simulink model "nms_3Dmodel_inv_wAnkleCPG"  (R2016b)
settings: Solver=ode3  StartTime=0.0  StopTime=tend  FixedStep=ts  RelTol=1e-3  EnableMultiTasking=on
InitFcn:
  | runScripts_inv;
values from neighbouring files (symbols this model uses):
  c = 0.05    [IID_nms_MechInit.m]    (also in nms_MechInit.m)
  c_jointstop = 0.3 / (pi/180)    (= 17.1887338539)    [IID_nms_MechInit.m]    (also in nms_MechInit.m)
  CPG_On = 1    [setCPGPar.m]    (also in setCPGPar_inv.m)
  CtrlPar_FP = [alpha0 alpha_cd alpha_cv]    [setCtrlPar.m]
  CtrlPar_FP_R = [R_hipR0 R_hipR_cd R_hipR_cv]    [setCtrlPar.m]
  CtrlPar_LL = l_clr    [setCtrlPar.m]
  CtrlPar_St = [StPreStim St_M1 St_M2 St_M3 St_M4 St_M5 St_M11]    [setCtrlPar.m]
  CtrlPar_St_R = [R_StPreStim R_St_M1 R_St_M3 R_St_M4]    [setCtrlPar.m]
  CtrlPar_Sw = [SwPreStim SwPhasePari SwPhaseParii SwCtrlPar_H SwCtrlPar_A      SwCtrlPar_Ki SwCtrlPar_Kii SwCtrlPar_Kiii SwCtrlPar_StP]    [setCtrlPar.m]
  CtrlPar_Sw_R = [R_SwPreStim R_Sw_M6]    [setCtrlPar.m]
  CtrlPar_theta0 = parBlCtrl(1)      *1*pi/180    [setCtrlPar.m]
  CtrlPar_Tr = [Tr_St_sup Tr_Sw]    [setCtrlPar.m]
  CtrlPar_Tr_R = [R_Tr_St_sup R_Tr_Sw]    [setCtrlPar.m]
  eref = 0.04    [IID_nms_MechInit.m]    (also in nms_MechInit.m)
  FmaxBFSH = 350    [nms_MechInit.m]
  FmaxGAS = 1500    [IID_nms_MechInit.m]    (also in nms_MechInit.m)
  FmaxGLU = 1500    [IID_nms_MechInit.m]    (also in nms_MechInit.m)
  FmaxHAB = 3000    [nms_MechInit.m]
  FmaxHAD = 4500    [nms_MechInit.m]
  FmaxHAM = 3000    [IID_nms_MechInit.m]    (also in nms_MechInit.m)
  FmaxHFL = 2000    [IID_nms_MechInit.m]    (also in nms_MechInit.m)
  FmaxRF = 1200    [nms_MechInit.m]
  FmaxSOL = 4000    [IID_nms_MechInit.m]    (also in nms_MechInit.m)
  FmaxTA = 800    [IID_nms_MechInit.m]    (also in nms_MechInit.m)
  FmaxVAS = 6000    [IID_nms_MechInit.m]    (also in nms_MechInit.m)
  init_a_tgt = 70*pi/180    (= 1.2217304764)    [setInitPar.m]
  init_a_tgtR = 90*pi/180    (= 1.57079632679)    [setInitPar.m]
  K = 5    [IID_nms_MechInit.m]    (also in nms_MechInit.m)
  leg_l = [D12_T D12_S]    [nms_MechInit.m]
  LongDelay = 0.020    (= 0.02)    [IID_setCtrlPar.m]    (also in nms_MechInit.m = 0.01)
  LongLoopDelay = 0.030    (= 0.03)    [nms_MechInit.m]
  loptBFSH = 0.12    [nms_MechInit.m]
  loptGAS = 0.05    [IID_nms_MechInit.m]    (also in nms_MechInit.m)
  loptGLU = 0.11    [IID_nms_MechInit.m]    (also in nms_MechInit.m)
  loptHAB = 0.09    [nms_MechInit.m]
  loptHAD = 0.10    (= 0.1)    [nms_MechInit.m]
  loptHAM = 0.10    (= 0.1)    [IID_nms_MechInit.m]    (also in nms_MechInit.m)
  loptHFL = 0.11    [IID_nms_MechInit.m]    (also in nms_MechInit.m)
  loptRF = 0.08    [nms_MechInit.m]
  loptSOL = 0.04    [IID_nms_MechInit.m]    (also in nms_MechInit.m)
  loptTA = 0.06    [IID_nms_MechInit.m]    (also in nms_MechInit.m)
  loptVAS = 0.08    [IID_nms_MechInit.m]    (also in nms_MechInit.m)
  lslackBFSH = 0.10    (= 0.1)    [nms_MechInit.m]
  lslackGAS = 0.40    (= 0.4)    [IID_nms_MechInit.m]    (also in nms_MechInit.m)
  lslackGLU = 0.13    [IID_nms_MechInit.m]    (also in nms_MechInit.m)
  lslackHAB = 0.07    [nms_MechInit.m]
  lslackHAD = 0.18    [nms_MechInit.m]
  lslackHAM = 0.31    [IID_nms_MechInit.m]    (also in nms_MechInit.m)
  lslackHFL = 0.10    (= 0.1)    [IID_nms_MechInit.m]    (also in nms_MechInit.m)
  lslackRF = 0.35    [nms_MechInit.m]
  lslackSOL = 0.26    [IID_nms_MechInit.m]    (also in nms_MechInit.m)
  lslackTA = 0.24    [IID_nms_MechInit.m]    (also in nms_MechInit.m)
  lslackVAS = 0.23    [IID_nms_MechInit.m]    (also in nms_MechInit.m)
  massBFSH = 2    [nms_MechInit.m]
  massGAS = 0.45    [IID_nms_MechInit.m]    (also in nms_MechInit.m)
  massGLU = 1.4    [IID_nms_MechInit.m]    (also in nms_MechInit.m)
  massHAB = 1.145    [nms_MechInit.m]
  massHAD = 1.91    [nms_MechInit.m]
  massHAM = 1.82    [IID_nms_MechInit.m]    (also in nms_MechInit.m)
  massHFL = 1.87    [IID_nms_MechInit.m]    (also in nms_MechInit.m)
  massRF = 1    [nms_MechInit.m]
  massSOL = 1.36    [IID_nms_MechInit.m]    (also in nms_MechInit.m)
  massTA = 0.29    [IID_nms_MechInit.m]    (also in nms_MechInit.m)
  massVAS = 2.91    [IID_nms_MechInit.m]    (also in nms_MechInit.m)
  MidDelay = 0.010    (= 0.01)    [IID_setCtrlPar.m]    (also in nms_MechInit.m = 0.005)
  N = 1.5    [IID_nms_MechInit.m]    (also in cmaes_parfor.m = size(x,1); nms_MechInit.m)
  phi12_LowLimit = 70*pi/180    (= 1.2217304764)    [IID_nms_MechInit.m]    (also in nms_MechInit.m)
  phi12_UpLimit = 130*pi/180    (= 2.26892802759)    [IID_nms_MechInit.m]    (also in nms_MechInit.m)
  phi23_UpLimit = 175*pi/180    (= 3.05432619099)    [IID_nms_MechInit.m]    (also in nms_MechInit.m)
  phi34_UpLimit = 230*pi/180    (= 4.01425727959)    [IID_nms_MechInit.m]    (also in nms_MechInit.m)
  phi34R_LowLimit = -15*pi/180    (= -0.261799387799)    [nms_MechInit.m]
  phi34R_UpLimit = 50*pi/180    (= 0.872664625997)    [nms_MechInit.m]
  phimaxGASa = 110*pi/180    (= 1.91986217719)    [IID_nms_MechInit.m]    (also in nms_MechInit.m = 1.74532925199)
  phimaxGASk = 140*pi/180    (= 2.44346095279)    [IID_nms_MechInit.m]    (also in nms_MechInit.m)
  phimaxRFk = 165*pi/180    (= 2.87979326579)    [nms_MechInit.m]
  phimaxSOL = 110*pi/180    (= 1.91986217719)    [IID_nms_MechInit.m]    (also in nms_MechInit.m = 1.74532925199)
  phimaxTA = 80*pi/180    (= 1.3962634016)    [IID_nms_MechInit.m]    (also in nms_MechInit.m)
  phimaxVAS = 165*pi/180    (= 2.87979326579)    [IID_nms_MechInit.m]    (also in nms_MechInit.m)
  phirefBFSH = 160*pi/180    (= 2.79252680319)    [nms_MechInit.m]
  phirefGASa = 80*pi/180    (= 1.3962634016)    [IID_nms_MechInit.m]    (also in nms_MechInit.m)
  phirefGASk = 165*pi/180    (= 2.87979326579)    [IID_nms_MechInit.m]    (also in nms_MechInit.m)
  phirefGLU = 150*pi/180    (= 2.61799387799)    [IID_nms_MechInit.m]    (also in nms_MechInit.m = 2.09439510239)
  phirefHAB = 10*pi/180    (= 0.174532925199)    [nms_MechInit.m]
  phirefHAD = 15*pi/180    (= 0.261799387799)    [nms_MechInit.m]
  phirefHAMh = 155*pi/180    (= 2.70526034059)    [IID_nms_MechInit.m]    (also in nms_MechInit.m = 2.61799387799)
  phirefHAMk = 180*pi/180    (= 3.14159265359)    [IID_nms_MechInit.m]    (also in nms_MechInit.m)
  phirefHFL = 180*pi/180    (= 3.14159265359)    [IID_nms_MechInit.m]    (also in nms_MechInit.m = 2.79252680319)
  phirefRFh = 170*pi/180    (= 2.96705972839)    [nms_MechInit.m]
  phirefRFk = 125*pi/180    (= 2.18166156499)    [nms_MechInit.m]
  phirefSOL = 80*pi/180    (= 1.3962634016)    [IID_nms_MechInit.m]    (also in nms_MechInit.m = 1.57079632679)
  phirefTA = 110*pi/180    (= 1.91986217719)    [IID_nms_MechInit.m]    (also in nms_MechInit.m)
  phirefVAS = 125*pi/180    (= 2.18166156499)    [IID_nms_MechInit.m]    (also in nms_MechInit.m = 2.09439510239)
  phiScaleGASa = acos(rGASamin/rGASamax)/(phiminGASa-phimaxGASa)    [nms_MechInit.m]
  phiScaleGASk = acos(rGASkmin/rGASkmax)/(phiminGASk-phimaxGASk)    [nms_MechInit.m]
  phiScaleRFk = acos(rRFkmin/rRFkmax)/(phiminRFk-phimaxRFk)    [nms_MechInit.m]
  phiScaleSOL = acos(rSOLmin/rSOLmax)/(phiminSOL-phimaxSOL)    [nms_MechInit.m]
  phiScaleTA = acos(rTAmin/rTAmax)/(phiminTA-phimaxTA)    [nms_MechInit.m]
  phiScaleVAS = acos(rVASmin/rVASmax)/(phiminVAS-phimaxVAS)    [nms_MechInit.m]
  rBFSH = 0.04    [nms_MechInit.m]
  rGASamax = 0.06    [nms_MechInit.m]
  rGASkmax = 0.05    [nms_MechInit.m]
  rGLU = 0.10    (= 0.1)    [IID_nms_MechInit.m]    (also in nms_MechInit.m = 0.08)
  rHAB = 0.06    [nms_MechInit.m]
  rHAD = 0.03    [nms_MechInit.m]
  rHAMh = 0.08    [IID_nms_MechInit.m]    (also in nms_MechInit.m)
  rHAMk = 0.05    [IID_nms_MechInit.m]    (also in nms_MechInit.m)
  rHFL = 0.10    (= 0.1)    [IID_nms_MechInit.m]    (also in nms_MechInit.m = 0.08)
  rhoBFSH = 0.7    [nms_MechInit.m]
  rhoGASa = 0.7    [IID_nms_MechInit.m]    (also in nms_MechInit.m)
  rhoGASk = 0.7    [IID_nms_MechInit.m]    (also in nms_MechInit.m)
  rhoGLU = 0.5    [IID_nms_MechInit.m]    (also in nms_MechInit.m)
  rhoHAB = 0.7    [nms_MechInit.m]
  rhoHAD = 1    [nms_MechInit.m]
  rhoHAMh = 0.7    [IID_nms_MechInit.m]    (also in nms_MechInit.m = 0.5)
  rhoHAMk = 0.7    [IID_nms_MechInit.m]    (also in nms_MechInit.m = 0.5)
  rhoHFL = 0.5    [IID_nms_MechInit.m]    (also in nms_MechInit.m)
  rhoRFh = 0.3    [nms_MechInit.m]
  rhoRFk = 0.5    [nms_MechInit.m]
  rhoSOL = 0.5    [IID_nms_MechInit.m]    (also in nms_MechInit.m)
  rhoTA = 0.7    [IID_nms_MechInit.m]    (also in nms_MechInit.m)
  ... (+55 more)
libraries: simulink_extras x30, nmc x30, simulink x22, NMCCPG_Library x13, powerlib_meascontrol x5
(part 1 of 12)
settings Model: SimulationMode=accelerator  Creator=Tycho  LastModifiedBy=brugtjh
settings DataIOCC: SignalLogging=off  SignalLoggingName=logout
settings OptimizationCC: LifeSpan=inf
settings DebuggingCC: AllowSymbolicDim=off  SFUnexpectedBacktrackingDiag=warning  SFNoUnconditionalDefaultTransitionDiag=warning  SFExecutionAtInitializationDiag=none
settings ModelReferenceCC: PropagateSignalLabelsOutOfModel=off
settings GRTTargetCC: TargetLangStandard=C89/C90 (ANSI)
settings ConfigComp: CovMetricSettings=dw  CovHtmlReporting=on  CovSaveCumulativeToWorkspaceVar=on  CovSaveSingleToWorkspaceVar=on  CovExternalEMLEnable=off

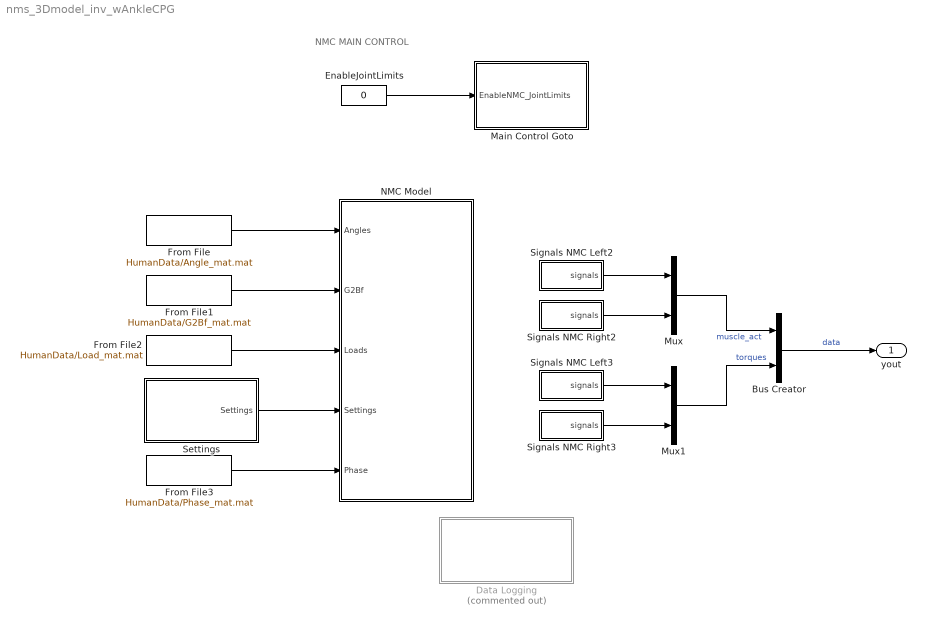
== system nms_3Dmodel_inv_wAnkleCPG ==
  note: NMC MAIN CONTROL
  Bus Creator : BusCreator  Inputs=2
  Data Logging : Subsystem  Commented=on
  EnableJointLimits : Constant  Value=0  OutDataTypeStr=double
      settings: OpenFcn=|
      | b = get_param(gcb,'value');
      | if (strcmp(b,'1')),
      |   set_param (gcb,'value','0');
      | else
      |   set_param(gcb,'value','1');
      | end;
  From File : FromFile  FileName=HumanData/Angle_mat.mat  SampleTime=0
  From File1 : FromFile  FileName=HumanData/G2Bf_mat.mat  SampleTime=0
  From File2 : FromFile  FileName=HumanData/Load_mat.mat  SampleTime=0
  From File3 : FromFile  FileName=HumanData/Phase_mat.mat  SampleTime=0
  Main Control Goto : Subsystem
  Mux : Mux  Inputs=2
  Mux1 : Mux  Inputs=2
  NMC Model : Subsystem
  Settings : Subsystem
  Signals NMC Left2 : Subsystem
  Signals NMC Left3 : Subsystem
  Signals NMC Right2 : Subsystem
  Signals NMC Right3 : Subsystem
  yout : Outport
  wires:
  Settings/1(Settings) -> NMC Model/4(Settings)
  EnableJointLimits/1 -> Main Control Goto/1(EnableNMC_JointLimits)
  From File/1 -> NMC Model/1(Angles)
  From File1/1 -> NMC Model/2(G2Bf)
  From File2/1 -> NMC Model/3(Loads)
  From File3/1 -> NMC Model/5(Phase)
  Signals NMC Right2/1(signals) -> Mux/2
  Signals NMC Left2/1(signals) -> Mux/1
  Signals NMC Left3/1(signals) -> Mux1/1
  Signals NMC Right3/1(signals) -> Mux1/2
  Mux/1 -> Bus Creator/1  "muscle_act"
  Mux1/1 -> Bus Creator/2  "torques"
  Bus Creator/1 -> yout/1  "data"

== system nms_3Dmodel_inv_wAnkleCPG/Data Logging ==
  note: Sensors
  note: Stance Info
  note: Muscle Activation
  note: Joint Torques
  note: Body Info
  note: Joint Torques (Passive)
  note: Muscle Power
  note: Angle of Attack
  Angles1 : Subsystem
  BodyInfo1 : Subsystem
  Joint Torques1 : Subsystem
  Joint TorquesPassive1 : Subsystem
  Joint TorquesTotal1 : Subsystem
  Loads1 : Subsystem
  M1 : Subsystem
  Muscle Activation2 : Subsystem
  Muscle Power1 : Subsystem
  Mux : Mux  Inputs=2
  Mux3 : Mux  Inputs=8
  Positions1 : Subsystem
  Selector2 : Selector  InputPortWidth=2  IndexOptions=Index vector (dialog)  Indices=[2]  OutputSizes=1
  Selector3 : Selector  InputPortWidth=2  IndexOptions=Index vector (dialog)  Indices=[2]  OutputSizes=1
  Sensors : Subsystem
  Signals NMC Left10 : Subsystem
  Signals NMC Left11 : Subsystem
  Signals NMC Left13 : Subsystem
  Signals NMC Left14 : Subsystem
  Signals NMC Left3 : Subsystem
  Signals NMC Left9 : Subsystem
  Signals NMC Right4 : Subsystem
  Signals NMC Right5 : Subsystem
  Signals NMC Right6 : Subsystem
  SignalsFromNMC_L1 : Subsystem  mask{LorR='L', Add=''}
      mask prompts: LorR "Right or Left"; Add "Addition"
      mask init:
      | blk = gcb;
      | set_param([gcb '/From'],'GotoTag',[LorR,'FmGLU',Add]);
      | set_param([gcb '/From1'],'GotoTag',[LorR,'FmHAM',Add]);
      | set_param([gcb '/From2'],'GotoTag',[LorR,'FmVAS',Add]);
      | set_param([gcb '/From3'],'GotoTag',[LorR,'LceBFSH',Add]);
      | set_param([gcb '/From4'],'GotoTag',[LorR,'FmGAS',Add]);
      | 
      | set_param([gcb '/From5'],'GotoTag',[LorR,'FmSOL',Add]);
      | set_param([gcb '/From6'],'GotoTag',[LorR,'LceTA',Add]);
      | set_param([gcb '/From7'],'GotoTag',[LorR,'LceRF',Add]);
      | set_param([gcb '/From8'],'GotoTag',[LorR,'VceRF',Add]);
      | set_param([gcb '/From9'],'GotoTag',[LorR,'LceHAM',Add]);
      | 
      | set_param([gcb '/From10'],'GotoTag',[LorR,'VceHAM',Add]);
      | set_param([gcb '/From11'],'GotoTag',[LorR,'VceVAS',Add]);
      | set_param([gcb '/From12'],'GotoTag',[LorR,'VceBFSH',Add]);
      | set_param([gcb '/From13'],'GotoTag',[LorR,'LceHFL',Add]);
      | set_param([gcb '/From14'],'GotoTag',[LorR,'LceGLU',Add]);
      | 
      | set_param([gcb '/From15'],'GotoTag',[LorR,'LceVAS',Add]);
      | set_param([gcb '/From16'],'GotoTag',[LorR,'FmHAB',Add]);
      | set_param([gcb '/From17'],'GotoTag',[LorR,'LceHAD',Add]);
      | set_param([gcb '/From18'],'GotoTag',[LorR,'LceHAB',Add]);
  SignalsFromNMC_L2 : Subsystem  mask{LorR='R', Add=''}
      mask prompts: LorR "Right or Left"; Add "Addition"
      mask init: same as nms_3Dmodel_inv_wAnkleCPG/Data Logging/SignalsFromNMC_L1
  StanceInfo1 : Subsystem
  Subsystem : Subsystem
  wires:
  SignalsFromNMC_L1/1(SigOut) -> Sensors/1(LC)
  SignalsFromNMC_L2/1(SigOut) -> Sensors/2(RC)
  Signals NMC Right5/1(signals) -> Muscle Activation2/2(R_MA)
  Signals NMC Left9/1(signals) -> Muscle Activation2/1(L_MA)
  Signals NMC Left10/1(signals) -> Joint TorquesTotal1/1(LTor)
  Signals NMC Right6/1(signals) -> Joint TorquesTotal1/2(RTor)
  Angles1/1(Angles) -> BodyInfo1/1(Angles)
  Positions1/1(Positions) -> BodyInfo1/2(Postitions)
  [LStance] -> StanceInfo1/1(LStance)
  [RStance] -> StanceInfo1/2(RStance)
  Loads1/1(Loads) -> BodyInfo1/3(Loads)
  [rotTrunk] -> Mux/1
  [theta] -> Mux/2
  Signals NMC Left11/1(signals) -> Joint TorquesPassive1/1(LTor)
  Signals NMC Right4/1(signals) -> Joint TorquesPassive1/2(RTor)
  Selector2/1 -> Mux3/1
  [front_dv_L] -> Selector2/1
  [L_M_TOT] -> Mux3/5
  [R_M_TOT] -> Mux3/6
  [L_M11_TOT] -> Mux3/3
  [R_M11_TOT] -> Mux3/4
  [front_dv_R] -> Selector3/1
  Selector3/1 -> Mux3/2
  Signals NMC Left13/1(signals) -> Muscle Power1/2(R_MA)
  Signals NMC Left14/1(signals) -> Muscle Power1/1(L_MA)
  Mux3/1 -> M1/1(M11)
  Mux/1 -> Subsystem/1(RotTrunk)
  [M11_Control] -> Mux3/8
  Signals NMC Left3/1(Target) -> Joint Torques1/1(Target)
  [front_v_est] -> Mux3/7

== system nms_3Dmodel_inv_wAnkleCPG/Main Control Goto ==
  EnableNMC_JointLimits : Inport
  tag scope: DisableNMC_JointLimitsIn=global
  wires:
  EnableNMC_JointLimits/1 -> [DisableNMC_JointLimitsIn]

== system nms_3Dmodel_inv_wAnkleCPG/NMC Model ==
  note: Data Distribution
  note: NMS model based on:
      | The nms_3Dmodel is a neuromechanical model of 3D human locomotion.
      | The details of the model are explained in:
      | S Song and H Geyer. "A neural circuitry that emphasizes spinal feedback
      | generates diverse behaviours of human locomotion." The Journal of physiology (2015).
      |
      | Muscle Actuation Layer:
      | The joints are actuated by 11 Hill-type muscles per leg.
      |
      | Neural Control Layer:
      | The muscles are controlled by local reflexes.
      |
      | Higher Control Layer:
      | The reflex pathways are modulated by the higher layer control.
  note: Neuromuscular Locomotion Model for Lopes
  note: DataStore for CPG
  Angles : Inport
  G2Bf : Inport  Port=2
  Loads : Inport  Port=3
  Settings : Inport  Port=4
  Phase : Inport  Port=5
  CPG : Subsystem
  Demux : Demux  Outputs=8
  Demux1 : Demux
  Demux2 : Demux  Outputs=2
  Demux4 : Demux
  Higher Control Layer (Supra Spinal Control) : Subsystem
  Muscle Actuation Layer : Subsystem
  Neural Control Layer (Spinal Cord Control) : Subsystem
  Rounding Function : Rounding  Operator=round
  Selector : Selector  InputPortWidth=12  IndexOptions=Index vector (dialog)  Indices=[1:4]  OutputSizes=1
  Selector1 : Selector  InputPortWidth=12  IndexOptions=Index vector (dialog)  Indices=[5:12]  OutputSizes=1
  data_l_st_freq : DataStoreMemory  DataStoreName=Freq_Ph1  ReadBeforeWriteMsg=warning  WriteAfterWriteMsg=warning  WriteAfterReadMsg=warning  InitialValue=FreqPL_Ph1  VectorParams1D=off  ShowAdditionalParam=off
  data_l_st_freq1 : DataStoreMemory  DataStoreName=Freq_Ph3  ReadBeforeWriteMsg=warning  WriteAfterWriteMsg=warning  WriteAfterReadMsg=warning  InitialValue=FreqPL_Ph3  VectorParams1D=off  ShowAdditionalParam=off
  data_l_st_shape : DataStoreMemory  DataStoreName=Shape_Ph1  ReadBeforeWriteMsg=warning  WriteAfterWriteMsg=warning  WriteAfterReadMsg=warning  InitialValue=ShapePL_Ph1  VectorParams1D=off  ShowAdditionalParam=off
  data_l_st_shape1 : DataStoreMemory  DataStoreName=Shape_Ph3  ReadBeforeWriteMsg=warning  WriteAfterWriteMsg=warning  WriteAfterReadMsg=warning  InitialValue=ShapePL_Ph3  VectorParams1D=off  ShowAdditionalParam=off
  data_l_sw_freq : DataStoreMemory  DataStoreName=Freq_Ph2  ReadBeforeWriteMsg=warning  WriteAfterWriteMsg=warning  WriteAfterReadMsg=warning  InitialValue=FreqPL_Ph2  VectorParams1D=off  ShowAdditionalParam=off
  data_l_sw_freq1 : DataStoreMemory  DataStoreName=Freq_Ph4  ReadBeforeWriteMsg=warning  WriteAfterWriteMsg=warning  WriteAfterReadMsg=warning  InitialValue=FreqPL_Ph4  VectorParams1D=off  ShowAdditionalParam=off
  data_l_sw_shape : DataStoreMemory  DataStoreName=Shape_Ph2  ReadBeforeWriteMsg=warning  WriteAfterWriteMsg=warning  WriteAfterReadMsg=warning  InitialValue=ShapePL_Ph2  VectorParams1D=off  ShowAdditionalParam=off
  data_l_sw_shape1 : DataStoreMemory  DataStoreName=Shape_Ph4  ReadBeforeWriteMsg=warning  WriteAfterWriteMsg=warning  WriteAfterReadMsg=warning  InitialValue=ShapePL_Ph4  VectorParams1D=off  ShowAdditionalParam=off
  etc : Subsystem
  tag scope: DisableNMC_JointLimits=global, LLLoad=global, Lphi12dphi12=global, Lphi23dphi23=global, Lphi34dphi34=global, Lphi34dphi34R=global, RLLoad=global, Rphi12dphi12=global, Rphi23dphi23=global, Rphi34dphi34=global, Rphi34dphi34R=global, dtheta=global, dthetaR=global, front_dv_L=global, front_dv_R=global, phase=global, side_dv_L=global, side_dv_R=global, theta=global, thetaR=global
  wires:
  Settings/1 -> [DisableNMC_JointLimits]
  Phase/1 -> Rounding Function/1
  Demux2/2 -> [RLLoad]
  Demux2/1 -> [LLLoad]
  Loads/1 -> Demux2/1
  G2Bf/1 -> Selector1/1, Selector/1
  Demux/4 -> [Lphi12dphi12]
  Demux/3 -> [Lphi23dphi23]
  Demux/2 -> [Lphi34dphi34R]
  Demux/8 -> [Rphi12dphi12]
  Demux/7 -> [Rphi23dphi23]
  Demux/6 -> [Rphi34dphi34R]
  Demux/5 -> [Rphi34dphi34]
  Demux/1 -> [Lphi34dphi34]
  Angles/1 -> Demux/1
  Demux4/1 -> [front_dv_L]
  Demux4/2 -> [front_dv_R]
  Demux4/3 -> [side_dv_L]
  Demux4/4 -> [side_dv_R]
  Demux1/4 -> [dthetaR]
  Demux1/3 -> [thetaR]
  Demux1/2 -> [dtheta]
  Demux1/1 -> [theta]
  Selector/1 -> Demux1/1
  Selector1/1 -> Demux4/1
  Rounding Function/1 -> [phase]

== system nms_3Dmodel_inv_wAnkleCPG/Settings ==
  Settings : Outport
  wires:
  [DisableNMC_JointLimitsIn] -> Settings/1

== system nms_3Dmodel_inv_wAnkleCPG/Signals NMC Left2 ==
  Mux : Mux  Inputs=11
  signals : Outport
  wires:
  Mux/1 -> signals/1
  [LStimHFL] -> Mux/1
  [LStimGLU] -> Mux/9
  [LStimVAS] -> Mux/3
  [LStimBFSH] -> Mux/7
  [LStimHAD] -> Mux/11
  [LStimSOL] -> Mux/5
  [LStimHAB] -> Mux/10
  [LStimHAM] -> Mux/8
  [LStimGAS] -> Mux/6
  [LStimTA] -> Mux/4
  [LStimRF] -> Mux/2

== system nms_3Dmodel_inv_wAnkleCPG/Signals NMC Left3 ==
  Mux : Mux
  signals : Outport
  wires:
  Mux/1 -> signals/1
  [LM34] -> Mux/1
  [LM23] -> Mux/3
  [LM12] -> Mux/4
  [LM34R] -> Mux/2

== system nms_3Dmodel_inv_wAnkleCPG/Signals NMC Right2 ==
  Mux : Mux  Inputs=11
  signals : Outport
  wires:
  [RStimRF] -> Mux/2
  [RStimTA] -> Mux/4
  [RStimGAS] -> Mux/6
  [RStimHAM] -> Mux/8
  [RStimHAB] -> Mux/10
  [RStimSOL] -> Mux/5
  [RStimHAD] -> Mux/11
  [RStimBFSH] -> Mux/7
  [RStimVAS] -> Mux/3
  [RStimGLU] -> Mux/9
  [RStimHFL] -> Mux/1
  Mux/1 -> signals/1

== system nms_3Dmodel_inv_wAnkleCPG/Signals NMC Right3 ==
  Mux : Mux
  signals : Outport
  wires:
  Mux/1 -> signals/1
  [RM34] -> Mux/1
  [RM23] -> Mux/3
  [RM12] -> Mux/4
  [RM34R] -> Mux/2

== system nms_3Dmodel_inv_wAnkleCPG/Data Logging/Angles1 ==
  Mux : Mux  Inputs=8
  Angles : Outport
  wires:
  [Rphi12dphi12] -> Mux/8
  [Lphi34dphi34] -> Mux/1
  [Rphi23dphi23] -> Mux/7
  [Lphi23dphi23] -> Mux/3
  [Rphi34dphi34R] -> Mux/6
  [Lphi34dphi34R] -> Mux/2
  [Lphi12dphi12] -> Mux/4
  [Rphi34dphi34] -> Mux/5
  Mux/1 -> Angles/1

== system nms_3Dmodel_inv_wAnkleCPG/Data Logging/BodyInfo1 ==
  Angles : Inport
  Postitions : Inport  Port=2
  Loads : Inport  Port=3
  Mux1 : Mux  Inputs=3
  To File8 : ToFile  Filename=Records/BodyInfo
  wires:
  Loads/1 -> Mux1/3
  Postitions/1 -> Mux1/2
  Mux1/1 -> To File8/1
  Angles/1 -> Mux1/1

== system nms_3Dmodel_inv_wAnkleCPG/Data Logging/Joint Torques1 ==
  Target : Inport
  To File12 : ToFile  Filename=Records/TargetAngle
  wires:
  Target/1 -> To File12/1

== system nms_3Dmodel_inv_wAnkleCPG/Data Logging/Joint TorquesPassive1 ==
  LTor : Inport
  RTor : Inport  Port=2
  To File12 : ToFile  Filename=Records/L_Tor_Passive
  To File9 : ToFile  Filename=Records/R_Tor_Passvie
  wires:
  RTor/1 -> To File9/1
  LTor/1 -> To File12/1

== system nms_3Dmodel_inv_wAnkleCPG/Data Logging/Joint TorquesTotal1 ==
  LTor : Inport
  RTor : Inport  Port=2
  To File12 : ToFile  Filename=Records/L_Tor
  To File9 : ToFile  Filename=Records/R_Tor
  wires:
  LTor/1 -> To File12/1
  RTor/1 -> To File9/1

== system nms_3Dmodel_inv_wAnkleCPG/Data Logging/Loads1 ==
  Mux : Mux  Inputs=2
  Loads : Outport
  wires:
  [LLLoad] -> Mux/2
  [RLLoad] -> Mux/1
  Mux/1 -> Loads/1

== system nms_3Dmodel_inv_wAnkleCPG/Data Logging/M1 ==
  M11 : Inport
  To File2 : ToFile  Filename=Records/M11
  wires:
  M11/1 -> To File2/1

== system nms_3Dmodel_inv_wAnkleCPG/Data Logging/Muscle Activation2 ==
  L_MA : Inport
  R_MA : Inport  Port=2
  To File1 : ToFile  Filename=Records/R_MA
  To File5 : ToFile  Filename=Records/L_MA
  wires:
  L_MA/1 -> To File5/1
  R_MA/1 -> To File1/1

== system nms_3Dmodel_inv_wAnkleCPG/Data Logging/Muscle Power1 ==
  L_MA : Inport
  R_MA : Inport  Port=2
  To File1 : ToFile  Filename=Records/R_Power
  To File5 : ToFile  Filename=Records/L_Power
  wires:
  L_MA/1 -> To File5/1
  R_MA/1 -> To File1/1

== system nms_3Dmodel_inv_wAnkleCPG/Data Logging/Positions1 ==
  Mux : Mux  Inputs=19
  Positions : Outport
  wires:
  [xyzRMBall] -> Mux/19
  [xyzRLBall] -> Mux/18
  [xyzRMHeel] -> Mux/17
  [xyzRLHeel] -> Mux/16
  [xyzLMBall] -> Mux/15
  [xyzLLBall] -> Mux/14
  [xyzLMHeel] -> Mux/13
  [xyzLLHeel] -> Mux/12
  [xyzTrunk] -> Mux/11
  [dxyzHAT] -> Mux/2
  [xyzHAT] -> Mux/1
  [dxyzRHip] -> Mux/10
  [xyzRHip] -> Mux/9
  [xyzLAnkle] -> Mux/3
  [xyzRKnee] -> Mux/8
  [dxyzLHip] -> Mux/6
  [xyzLHip] -> Mux/5
  [xyzLKnee] -> Mux/4
  [xyzRAnkle] -> Mux/7
  Mux/1 -> Positions/1

== system nms_3Dmodel_inv_wAnkleCPG/Data Logging/Sensors ==
  LC : Inport
  RC : Inport  Port=2
  To File19 : ToFile  Filename=Records/L_Clean
  To File20 : ToFile  Filename=Records/R_Clean
  wires:
  RC/1 -> To File20/1
  LC/1 -> To File19/1

== system nms_3Dmodel_inv_wAnkleCPG/Data Logging/Signals NMC Left10 ==
  Mux : Mux
  signals : Outport
  wires:
  [LM34R] -> Mux/2
  [LM12] -> Mux/4
  [LM23] -> Mux/3
  [LM34] -> Mux/1
  Mux/1 -> signals/1

== system nms_3Dmodel_inv_wAnkleCPG/Data Logging/Signals NMC Left11 ==
  Mux : Mux
  signals : Outport
  wires:
  Mux/1 -> signals/1
  [LHipStop] -> Mux/1
  [LKneeStop] -> Mux/3
  [LAnkleStop] -> Mux/4
  [LHipRStop] -> Mux/2

== system nms_3Dmodel_inv_wAnkleCPG/Data Logging/Signals NMC Left13 ==
  Mux : Mux  Inputs=11
  signals : Outport
  wires:
  Mux/1 -> signals/1
  [REnergyHFL] -> Mux/1
  [REnergyGLU] -> Mux/9
  [REnergyVAS] -> Mux/3
  [REnergyBFSH] -> Mux/7
  [REnergyHAD] -> Mux/11
  [REnergySOL] -> Mux/5
  [REnergyHAB] -> Mux/10
  [REnergyHAM] -> Mux/8
  [REnergyGAS] -> Mux/6
  [REnergyTA] -> Mux/4
  [REnergyRF] -> Mux/2

== system nms_3Dmodel_inv_wAnkleCPG/Data Logging/Signals NMC Left14 ==
  Mux : Mux  Inputs=11
  signals : Outport
  wires:
  [LEnergyRF] -> Mux/2
  [LEnergyTA] -> Mux/4
  [LEnergyGAS] -> Mux/6
  [LEnergyHAM] -> Mux/8
  [LEnergyHAB] -> Mux/10
  [LEnergySOL] -> Mux/5
  [LEnergyHAD] -> Mux/11
  [LEnergyBFSH] -> Mux/7
  [LEnergyVAS] -> Mux/3
  [LEnergyGLU] -> Mux/9
  [LEnergyHFL] -> Mux/1
  Mux/1 -> signals/1

== system nms_3Dmodel_inv_wAnkleCPG/Data Logging/Signals NMC Left3 ==
  Mux : Mux
  Target : Outport
  wires:
  Mux/1 -> Target/1
  [Lalpha_tgt] -> Mux/1
  [LhipR_tgt] -> Mux/3
  [RhipR_tgt] -> Mux/4
  [Ralpha_tgt] -> Mux/2

== system nms_3Dmodel_inv_wAnkleCPG/Data Logging/Signals NMC Left9 ==
  Mux : Mux  Inputs=11
  signals : Outport
  wires:
  [LStimRF] -> Mux/2
  [LStimTA] -> Mux/4
  [LStimGAS] -> Mux/6
  [LStimHAM] -> Mux/8
  [LStimHAB] -> Mux/10
  [LStimSOL] -> Mux/5
  [LStimHAD] -> Mux/11
  [LStimBFSH] -> Mux/7
  [LStimVAS] -> Mux/3
  [LStimGLU] -> Mux/9
  [LStimHFL] -> Mux/1
  Mux/1 -> signals/1

== system nms_3Dmodel_inv_wAnkleCPG/Data Logging/Signals NMC Right4 ==
  Mux : Mux
  signals : Outport
  wires:
  Mux/1 -> signals/1
  [RHipStop] -> Mux/1
  [RKneeStop] -> Mux/3
  [RAnkleStop] -> Mux/4
  [RHipStopR] -> Mux/2

== system nms_3Dmodel_inv_wAnkleCPG/Data Logging/Signals NMC Right5 ==
  Mux : Mux  Inputs=11
  signals : Outport
  wires:
  Mux/1 -> signals/1
  [RStimHFL] -> Mux/1
  [RStimGLU] -> Mux/9
  [RStimVAS] -> Mux/3
  [RStimBFSH] -> Mux/7
  [RStimHAD] -> Mux/11
  [RStimSOL] -> Mux/5
  [RStimHAB] -> Mux/10
  [RStimHAM] -> Mux/8
  [RStimGAS] -> Mux/6
  [RStimTA] -> Mux/4
  [RStimRF] -> Mux/2

== system nms_3Dmodel_inv_wAnkleCPG/Data Logging/Signals NMC Right6 ==
  Mux : Mux
  signals : Outport
  wires:
  [RM34R] -> Mux/2
  [RM12] -> Mux/4
  [RM23] -> Mux/3
  [RM34] -> Mux/1
  Mux/1 -> signals/1

== system nms_3Dmodel_inv_wAnkleCPG/Data Logging/SignalsFromNMC_L1 ==
  Mux1 : Mux  Inputs=19
  SigOut : Outport
  wires:
  [LLceVAS] -> Mux1/16
  [LVceHAM] -> Mux1/11
  Mux1/1 -> SigOut/1
  [LVceVAS] -> Mux1/12
  [LLceRF] -> Mux1/8
  [LLceGLU] -> Mux1/15
  [LFmGAS] -> Mux1/5
  [LVceBFSH] -> Mux1/13
  [LLceHAD] -> Mux1/18
  [LVceRF] -> Mux1/9
  [LLceBFSH] -> Mux1/4
  [LFmGLU] -> Mux1/1
  [LFmSOL] -> Mux1/6
  [LLceHFL] -> Mux1/14
  [LFmVAS] -> Mux1/3
  [LLceTA] -> Mux1/7
  [LFmHAM] -> Mux1/2
  [LLceHAM] -> Mux1/10
  [LFmHAB] -> Mux1/17
  [LLceHAB] -> Mux1/19

== system nms_3Dmodel_inv_wAnkleCPG/Data Logging/SignalsFromNMC_L2 ==
  Mux1 : Mux  Inputs=19
  SigOut : Outport
  wires:
  [RLceHAB] -> Mux1/19
  [RFmHAB] -> Mux1/17
  [RLceHAM] -> Mux1/10
  [RFmHAM] -> Mux1/2
  [RLceTA] -> Mux1/7
  [RFmVAS] -> Mux1/3
  [RLceHFL] -> Mux1/14
  [RFmSOL] -> Mux1/6
  [RFmGLU] -> Mux1/1
  [RLceBFSH] -> Mux1/4
  [RVceRF] -> Mux1/9
  [RLceHAD] -> Mux1/18
  [RVceBFSH] -> Mux1/13
  [RFmGAS] -> Mux1/5
  [RLceGLU] -> Mux1/15
  [RLceRF] -> Mux1/8
  [RVceVAS] -> Mux1/12
  Mux1/1 -> SigOut/1
  [RVceHAM] -> Mux1/11
  [RLceVAS] -> Mux1/16

== system nms_3Dmodel_inv_wAnkleCPG/Data Logging/StanceInfo1 ==
  LStance : Inport
  RStance : Inport  Port=2
  Mux4 : Mux  Inputs=2
  To File4 : ToFile  Filename=Records/StanceSig
  wires:
  LStance/1 -> Mux4/1
  RStance/1 -> Mux4/2
  Mux4/1 -> To File4/1

== system nms_3Dmodel_inv_wAnkleCPG/Data Logging/Subsystem ==
  RotTrunk : Inport
  To File8 : ToFile  Filename=Records/rotTrunk
  wires:
  RotTrunk/1 -> To File8/1

== system nms_3Dmodel_inv_wAnkleCPG/NMC Model/CPG ==
  note: CPG State Observer
      | Learning Center
      | Learns the signals of all sensors
      | If signals are prelearned, only loads the signals
      |
      | CPG Output
      | Estimates rate of change (roc at all instances of various time model
      | Becomes active after signals are saved or loaded
      |
      | Saver
      | Saves signals to workspace after learning is done
      |
      | Etc
      | Creates signals necessary in CPG model
  CPG Output : Subsystem
  Etc : Subsystem
  Learning center : Subsystem

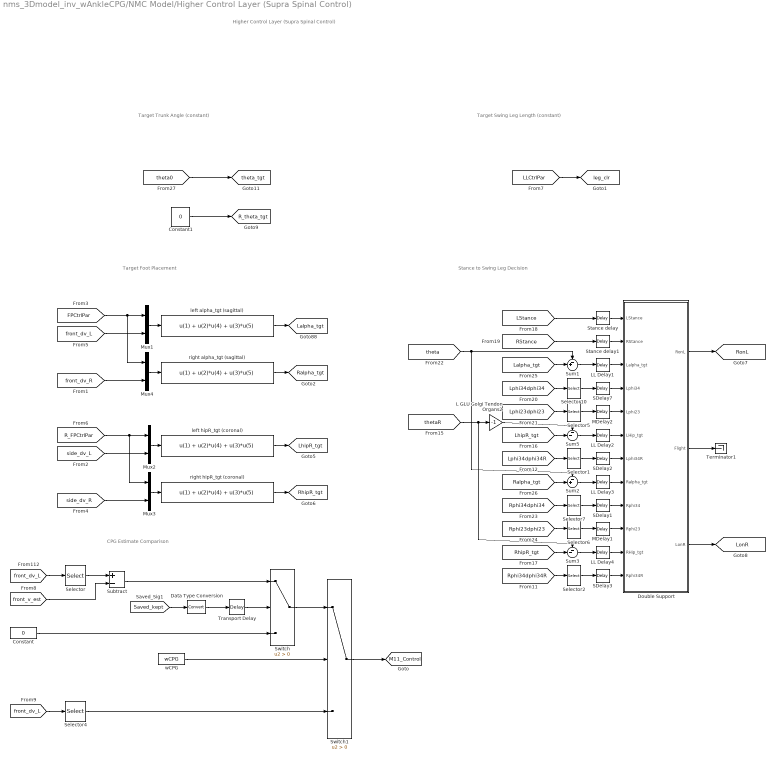
== system nms_3Dmodel_inv_wAnkleCPG/NMC Model/Higher Control Layer (Supra Spinal Control) ==
  note: Higher Control Layer
      | (Supra Spinal Control)
  note: Target Trunk Angle
      | (constant)
  note: Stance to Swing Leg Decision
  note: Target Swing Leg Length
      | (constant)
  note: Target Foot Placement
  note: CPG Estimate Comparison
  Constant : Constant  Value=0
  Constant1 : Constant  Value=0
  Data Type Conversion : DataTypeConversion
  Double Support : Subsystem
  L GLU Golgi Tendon Organs2 : Gain  Gain=-1
  LL Delay1 : TransportDelay  DelayTime=LongLoopDelay/2  InitialOutput=init_a_tgt
  LL Delay2 : TransportDelay  DelayTime=LongLoopDelay/2
  LL Delay3 : TransportDelay  DelayTime=LongLoopDelay/2  InitialOutput=init_a_tgt
  LL Delay4 : TransportDelay  DelayTime=LongLoopDelay/2
  MDelay1 : TransportDelay  DelayTime=MidDelay
  MDelay2 : TransportDelay  DelayTime=MidDelay
  Mux{1..4} (4 alike) : Mux  Inputs=2
  SDelay{1..3,7} (4 alike) : TransportDelay  DelayTime=ShortDelay
  Selector : Selector  InputPortWidth=2  IndexOptions=Index vector (dialog)  Indices=[2]  OutputSizes=1
  Selector{1..2,5..7,10} (6 alike) : Selector  InputPortWidth=2  IndexOptions=Index vector (dialog)  Indices=1  OutputSizes=1
  Selector4 : Selector  InputPortWidth=2  IndexOptions=Index vector (dialog)  Indices=[2]  OutputSizes=1
  Stance delay : TransportDelay  DelayTime=MidDelay
  Stance delay1 : TransportDelay  DelayTime=MidDelay
  Subtract : Sum  Inputs=+-
  Sum1 : Sum  Inputs=-+|
  Sum2 : Sum  Inputs=-+|
  Sum3 : Sum  Inputs=--|
  Sum5 : Sum  Inputs=--|
  Switch : Switch  Criteria=u2 > Threshold
  Switch1 : Switch  Criteria=u2 > Threshold
  Terminator1 : Terminator
  Transport Delay : TransportDelay  DelayTime=0.1
  left alpha_tgt (sagittal) : Fcn  Expr=u(1) + u(2)*u(4) + u(3)*u(5)
  left hipR_tgt (coronal) : Fcn  Expr=u(1) + u(2)*u(4) + u(3)*u(5)
  right alpha_tgt (sagittal) : Fcn  Expr=u(1) + u(2)*u(4) + u(3)*u(5)
  right hipR_tgt (coronal) : Fcn  Expr=u(1) + u(2)*u(4) + u(3)*u(5)
  wCPG : Constant  Value=wCPG
  tag scope: Lalpha_tgt=global, LhipR_tgt=global, LonR=global, M11_Control=global, R_theta_tgt=global, Ralpha_tgt=global, RhipR_tgt=global, RonL=global, leg_clr=global, theta_tgt=global
  wires:
  [side_dv_R] -> Mux3/2
  [side_dv_L] -> Mux2/2
  [R_FPCtrlPar] -> Mux2/1, Mux3/1
  Mux3/1 -> right hipR_tgt (coronal)/1
  Mux2/1 -> left hipR_tgt (coronal)/1
  [front_dv_R] -> Mux4/2
  Mux4/1 -> right alpha_tgt (sagittal)/1
  [front_dv_L] -> Mux1/2
  [FPCtrlPar] -> Mux1/1, Mux4/1
  Mux1/1 -> left alpha_tgt (sagittal)/1
  Constant1/1 -> [R_theta_tgt]
  [theta0] -> [theta_tgt]
  [RhipR_tgt] -> Sum3/2
  Sum3/1 -> LL Delay4/1
  LL Delay4/1 -> Double Support/11(RHip_tgt)
  SDelay3/1 -> Double Support/12(Rphi34R)
  Selector2/1 -> SDelay3/1
  [Rphi34dphi34R] -> Selector2/1
  L GLU Golgi Tendon Organs2/1 -> Sum5/1
  [thetaR] -> Sum3/1, L GLU Golgi Tendon Organs2/1
  [LhipR_tgt] -> Sum5/2
  Sum5/1 -> LL Delay2/1
  LL Delay2/1 -> Double Support/6(LHip_tgt)
  SDelay2/1 -> Double Support/7(Lphi34R)
  Selector1/1 -> SDelay2/1
  [Lphi34dphi34R] -> Selector1/1
  Sum2/1 -> LL Delay3/1
  [Ralpha_tgt] -> Sum2/2
  [theta] -> Sum2/1, Sum1/1
  [Lalpha_tgt] -> Sum1/2
  Sum1/1 -> LL Delay1/1
  MDelay1/1 -> Double Support/10(Rphi23)
  MDelay2/1 -> Double Support/5(Lphi23)
  SDelay1/1 -> Double Support/9(Rphi34)
  SDelay7/1 -> Double Support/4(Lphi34)
  LL Delay3/1 -> Double Support/8(Ralpha_tgt)
  LL Delay1/1 -> Double Support/3(Lalpha_tgt)
  Double Support/2(Flight) -> Terminator1/1
  [RStance] -> Stance delay1/1
  [LStance] -> Stance delay/1
  Double Support/1(RonL) -> [RonL]
  Stance delay1/1 -> Double Support/2(RStance)
  Stance delay/1 -> Double Support/1(LStance)
  Double Support/3(LonR) -> [LonR]
  Selector6/1 -> MDelay1/1
  Selector7/1 -> SDelay1/1
  [Rphi23dphi23] -> Selector6/1
  [Rphi34dphi34] -> Selector7/1
  Selector5/1 -> MDelay2/1
  Selector10/1 -> SDelay7/1
  [Lphi23dphi23] -> Selector5/1
  [Lphi34dphi34] -> Selector10/1
  [LLCtrlPar] -> [leg_clr]
  right hipR_tgt (coronal)/1 -> [RhipR_tgt]
  left hipR_tgt (coronal)/1 -> [LhipR_tgt]
  right alpha_tgt (sagittal)/1 -> [Ralpha_tgt]
  left alpha_tgt (sagittal)/1 -> [Lalpha_tgt]
  [front_dv_L] -> Selector/1
  Selector/1 -> Subtract/1
  [front_v_est] -> Subtract/2
  Subtract/1 -> Switch/1
  [Saved_kept] -> Data Type Conversion/1
  Switch/1 -> Switch1/1
  Transport Delay/1 -> Switch/2
  Constant/1 -> Switch/3
  Data Type Conversion/1 -> Transport Delay/1
  [front_dv_L] -> Selector4/1
  Selector4/1 -> Switch1/3
  Switch1/1 -> [M11_Control]
  wCPG/1 -> Switch1/2
